simulink model "sim_feedback_lin"  (R2015a)
settings: Solver=ode45  StartTime=0.0  StopTime=5  RelTol=1e-3
values from neighbouring files (symbols this model uses):
  A = [0 0 1 0 ... (first row only)    [MAIN_feedback_lin.m]    (also in MAIN_finite_lqr.m)
  B = [0 0 ... (first row only)    [MAIN_feedback_lin.m]    (also in MAIN_finite_lqr.m)
  K = -lqr(A,B,q,r)    [MAIN_feedback_lin.m]    (also in finite_lqr.m = R\B'*P)
  m = size(B, 2)    [MAIN_feedback_lin.m]    (also in MAIN_finite_lqr.m)
  n = size(A, 1)    [MAIN_feedback_lin.m]    (also in MAIN_finite_lqr.m; feedback_lin_finite_lqr.m = 50)
  u_star = -B' * A * x_star    [MAIN_feedback_lin.m]    (also in MAIN_finite_lqr.m)
  x_star = [theta_star; 0; 0]    [MAIN_feedback_lin.m]    (also in MAIN_finite_lqr.m)
settings Model: Creator=Ian  LastModifiedBy=Ian

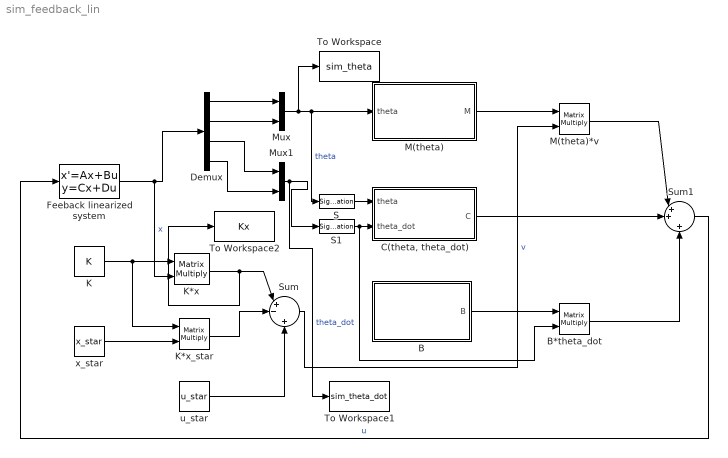
== system sim_feedback_lin ==
  B : MATLAB Function  TreatAsAtomicUnit=on
  B*theta_dot : Product  Multiplication=Matrix(*)
  "C(theta, theta_dot)" : MATLAB Function  TreatAsAtomicUnit=on
  Demux : Demux
  Feeback linearized system : StateSpace  A=A  B=B  C=eye(n)  D=zeros(n,m)  X0=[pi/2 pi/2 0 0]
  K : Constant  Value=K
  K*x : Product  Multiplication=Matrix(*)
  K*x_star : Product  Multiplication=Matrix(*)
  M(theta) : MATLAB Function  TreatAsAtomicUnit=on
  M(theta)*v : Product  Multiplication=Matrix(*)
  Mux : Mux  Inputs=2
  Mux1 : Mux  Inputs=2
  S : SignalSpecification  Dimensions=[2 1]
  S1 : SignalSpecification  Dimensions=[2 1]
  Sum : Sum  Inputs=|+-|+
  Sum1 : Sum  Inputs=|++|+
  To Workspace : ToWorkspace  VariableName=sim_theta  SaveFormat=Timeseries  SampleTime=-1
  To Workspace1 : ToWorkspace  VariableName=sim_theta_dot  SaveFormat=Timeseries  SampleTime=-1
  To Workspace2 : ToWorkspace  VariableName=Kx  SaveFormat=Timeseries  SampleTime=-1
  u_star : Constant  Value=u_star
  x_star : Constant  Value=x_star
  wires:
  Feeback linearized system/1 -> K*x/2, Demux/1  "x"
  Demux/1 -> Mux/1
  Demux/2 -> Mux/2
  Mux/1 -> To Workspace/1, M(theta)/1(theta), S/1  "theta"
  Demux/3 -> Mux1/1
  Demux/4 -> Mux1/2
  Mux1/1 -> To Workspace1/1, S1/1  "theta_dot"
  K/1 -> K*x_star/1, K*x/1
  x_star/1 -> K*x_star/2
  K*x/1 -> To Workspace2/1, Sum/1
  K*x_star/1 -> Sum/2
  u_star/1 -> Sum/3
  Sum/1 -> M(theta)*v/2  "v"
  M(theta)/1(M) -> M(theta)*v/1
  B/1(B) -> B*theta_dot/1
  M(theta)*v/1 -> Sum1/1
  "C(theta, theta_dot)"/1(C) -> Sum1/2
  B*theta_dot/1 -> Sum1/3
  Sum1/1 -> Feeback linearized system/1  "u"
  S/1 -> "C(theta, theta_dot)"/1(theta)
  S1/1 -> B*theta_dot/2, "C(theta, theta_dot)"/2(theta_dot)

== matlab function sim_feedback_lin/C(theta, theta_dot) ==
  data: theta input; C output; theta_dot input
function C = sim_coriolis_mtx(theta, theta_dot)

C = coriolis_mtx(theta, theta_dot);

== matlab function sim_feedback_lin/M(theta) ==
  data: theta input; M output
function M = sim_intertia_mtx(theta)

M = inertia_mtx(theta);

== matlab function sim_feedback_lin/B ==
  data: B output
function B = sim_joint_friction_mtx

B = joint_friction_mtx();
